simulink model "BLDCmotor_FOC_R2017b_fixdt"  (R2025a)
settings: Solver=FixedStepDiscrete  StartTime=0  StopTime=0.5  FixedStep=Ts  MaxStep=1e-6  RelTol=1e-6  AbsTol=1e-6  EnableMultiTasking=on
PreLoadFcn:
  | addpath(pwd);
  | addpath(genpath('01_Libraries'));
  | addpath(genpath('02_Figures'));
  | addpath(genpath('03_CreateParamTable'));
InitFcn:
  | init_model;
values from neighbouring files (symbols this model uses):
  a_cpr = 65535    [init_model.m]
  a_elecAngle = 60    [init_model.m]
  a_elecoffset = a_elecPeriod/12    (= 30)    [init_model.m]
  a_elecPeriod = 360    [init_model.m]
  a_fcpr = 1/65535    (= 1.52590218967e-05)    [init_model.m]
  a_mechoffset = a_elecoffset/n_polePairs    (= 5)    [init_model.m]
  a_phaAdvMax = 25    [init_model.m]
  b_angleMeasEna = 1    [init_model.m]
  b_cruiseCtrlEna = 0    [init_model.m]
  b_diagEna = 0    [init_model.m]
  b_fieldWeakEna = 0    [init_model.m]
  cf_currFilt = 0.692    [init_model.m]
  cf_idKi = Ki / (f_ctrl)    (= 0.00409061543436)    [init_model.m]
  cf_idKp = Kp    (= 0.0523598775598)    [init_model.m]
  cf_iqKi = Ki / (f_ctrl)    (= 0.00409061543436)    [init_model.m]
  cf_iqKiLimProt = 60 / (f_ctrl)    (= 0.00375)    [init_model.m]
  cf_iqKp = Kp    (= 0.0523598775598)    [init_model.m]
  cf_KbLimProt = Simulink.Parameter    [init_model.m]
  cf_nKi = 20.4 / (f_ctrl)    (= 0.001275)    [init_model.m]
  cf_nKiLimProt = 20 / (f_ctrl)    (= 0.00125)    [init_model.m]
  cf_nKp = 1.18    [init_model.m]
  cf_speedCoef = round(f_ctrl * a_mechAngle * (pi/180) * (30/pi))    [init_model.m]
  CTRL_FOC = 2    [init_model.m]
  CTRL_SIN = 1    [init_model.m]
  dV_openRate = 1000 / (f_ctrl)    (= 0.0625)    [init_model.m]
  dz_cntTrnsDetHi = 40    [init_model.m]
  dz_cntTrnsDetLo = 20    [init_model.m]
  ff_gain = ((r_motn / i_sca) * ((GD32_Vd_max_margin) / v_bus))    (= 0.338958333333)    [init_model.m]
  GD32_Vd_max_margin = GD32_Vd_max - V_margin    (= 1627)    [init_model.m]
  GD32_Vq_max_M1 = sqrt(GD32_Vd_max_margin^2 - GD32_Vq_max_XA.^2)    [init_model.m]
  i_max = i_max * i_sca    (= 500)    [init_model.m]
  id_fieldWeakMax = 5 * i_sca    (= 250)    [init_model.m]
  iq_maxSca_M1 = sqrt(1 - iq_maxSca_XA.^2)    [init_model.m]
  mcu_model = GD32F103    (= 1)    [init_model.m]
  n_commAcvLo = 15    [init_model.m]
  n_commDeacvHi = 30    [init_model.m]
  n_cruiseMotTgt = 0    [init_model.m]
  n_fieldWeakAuthHi = 300    [init_model.m]
  n_fieldWeakAuthLo = 100    [init_model.m]
  n_max = 1950    [init_model.m]
  n_polePairs = 6    [init_model.m]
  n_stdStillDet = 3    [init_model.m]
  OPEN_MODE = 0    [init_model.m]
  r_cos_M1 = cos((a_elecAngle_XA + a_elecPeriod/12)*(pi/180))    [init_model.m]
  r_errInpTgtThres = 600    [init_model.m]
  r_fieldWeakHi = 1000    [init_model.m]
  r_fieldWeakLo = 750    [init_model.m]
  r_motn = r_mot/2    (= 0.25)    [init_model.m]
  r_sin3PhaA_M1 = sin3Arm + A*r_sinPhaA_M1    [init_model.m]
  r_sin3PhaB_M1 = sin3Arm + A*r_sinPhaB_M1    [init_model.m]
  r_sin3PhaC_M1 = sin3Arm + A*r_sinPhaC_M1    [init_model.m]
  r_sin_M1 = sin((a_elecAngle_XA + a_elecPeriod/12)*(pi/180))    [init_model.m]
  SPD_MODE = 2    [init_model.m]
  STM32_Vd_max_margin = STM32_Vd_max - V_margin    (= 940)    [init_model.m]
  STM32_Vq_max_M1 = sqrt(STM32_Vd_max_margin^2 - STM32_Vq_max_XA.^2)    [init_model.m]
  t_errDequal = 1.80 * f_ctrl    (= 28800)    [init_model.m]
  t_errQual = 0.24 * f_ctrl    (= 3840)    [init_model.m]
  tgt_scale = 2047    [init_model.m]
  TRQ_MODE = 3    [init_model.m]
  Ts = 5e-6    (= 5e-06)    [init_model.m]
  Ts_ctrl = 6e-5    (= 6e-05)    [init_model.m]
  v_bus = 24    [init_model.m]
  vec_hallToPos = [0 2 0 1 4 3 5 0]    [init_model.m]
  VLT_MODE = 1    [init_model.m]
  z_commutMap_M1 = [-1 -1  0  1  1  0 ... (first row only)    [init_model.m]
  z_ctrlModReq = TRQ_MODE    (= 3)    [init_model.m]
  z_ctrlTypSel = CTRL_FOC    (= 2)    [init_model.m]
  z_maxCntRst = 2000    [init_model.m]
  z_selPhaCurMeasABC = 2    [init_model.m]
undefined symbols (not defined in the file or in its folder): BLDCmotor_FOC_R2017b_fixdt, DiscIntNeverNeededParam, DWORK0, DWORK1, DWORK2, DWORK3, powergui, spspowerguiLib
libraries: BLDC_controller_Lib x18, simulink x13, prociolib x6, eePwmGenerator x6, eePwmGeneratorMultilevel x3, mcbpositiondecoderlib x2, slpidlib x2, spsControlledVoltageSourceLib x1, spsMultimeterLib x1, spsPermanentMagnetSynchronousMachineLib x1, spsUniversalBridgeLib x1, spsVoltageMeasurementLib x1
(part 5 of 6)

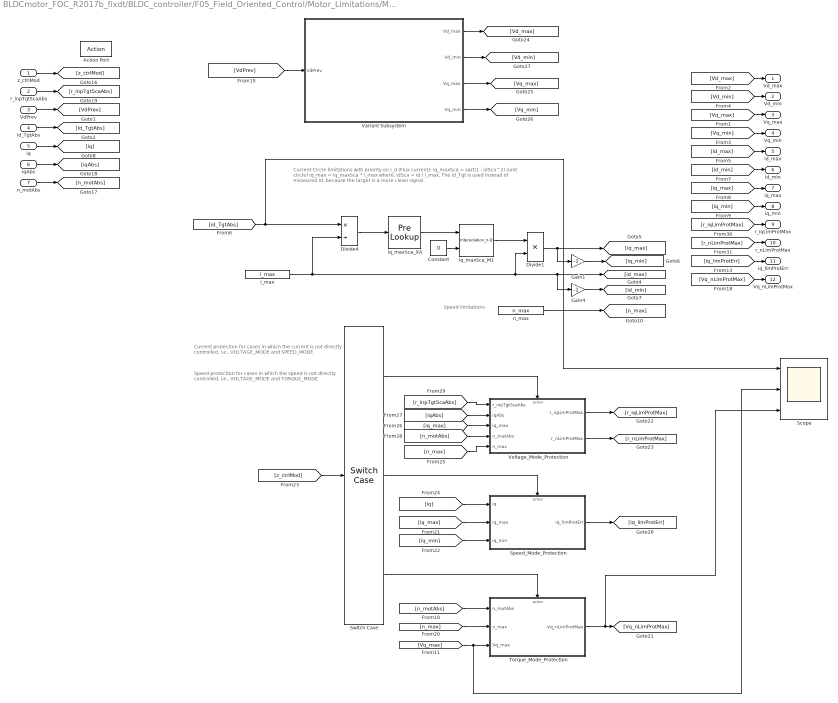
== system BLDCmotor_FOC_R2017b_fixdt/BLDC_controller/F05_Field_Oriented_Control/Motor_Limitations/Motor_Limitations_Enabled ==
  note: Current Circle limitations with priority on i_d (Flux current):
      | iq_maxSca = sqrt(1 - idSca^2) (unit circle)
      | iq_max = iq_maxSca * i_max
      |
      | where, idSca = id / i_max,
      |
      | The id_Tgt is used instead of measured id, because the target is a more clean signal.
  note: Speed limitations
  note: Current protection
      | for cases in which the current is not directly controlled, i.e., VOLTAGE_MODE and SPEED_MODE
  note: Speed protection
      | for cases in which the speed is not directly controlled, i.e., VOLTAGE_MODE and TORQUE_MODE
  z_ctrlMod : Inport
  r_inpTgtScaAbs : Inport  Port=2
  VdPrev : Inport  Port=3
  id_TgtAbs : Inport  Port=4
  iq : Inport  Port=5
  iqAbs : Inport  Port=6
  n_motAbs : Inport  Port=7
  Action Port : ActionPort  ActionPortLabel=if(u1 == CTRL_FOC)
  Constant : Constant  Value=0  OutDataTypeStr=int8
  Divide1 : Product  Inputs=**  OutDataTypeStr=fixdt(1,16,4)  RndMeth=Simplest
  Divide4 : Product  Inputs=*/  OutDataTypeStr=fixdt(0,16,16)  RndMeth=Simplest  SaturateOnIntegerOverflow=on
  Gain1 : Gain  Tag=struct('comment',struct('text','','placement',1),'logdata',struct('maxnumvals',inf,'plotchannels',[],'loggingmode',3,'channels',1),'output',struct('variable','','description','','name','$S_$B','width',1,'address','','max',NaN,'min',NaN,'class','default','type','CONTINUOUS','scaling','','lsb',1,'offset',0,'arb',0,'freeze',1,'unit','','autoscalingmode',1,'lowerheadroom',1,'upperheadroom',1,'headroomunit','bit','keepdatatype',1,'checkmin',0,'checkmax',0,'castoutput',0,'show',0),'gain',struct('variable','','description','','name','$S_$B_gain','width',1,'address','','max',NaN,'min',NaN,'class','default','type','CONTINUOUS','scaling','','lsb',1,'offset',0,'arb',0,'freeze',1,'unit','','keepdatatype',1,'value','1','scalar',0,'tolerance',1),'scalingvalid',0,'date',730486)  Gain=-1  RndMeth=Zero  OutDataTypeStr=Inherit: Same as input  ParamDataTypeStr=Inherit: Same as input
  Gain4 : Gain  Tag=struct('comment',struct('text','','placement',1),'logdata',struct('maxnumvals',inf,'plotchannels',[],'loggingmode',3,'channels',1),'output',struct('variable','','description','','name','$S_$B','width',1,'address','','max',NaN,'min',NaN,'class','default','type','CONTINUOUS','scaling','','lsb',1,'offset',0,'arb',0,'freeze',1,'unit','','autoscalingmode',1,'lowerheadroom',1,'upperheadroom',1,'headroomunit','bit','keepdatatype',1,'checkmin',0,'checkmax',0,'castoutput',0,'show',0),'gain',struct('variable','','description','','name','$S_$B_gain','width',1,'address','','max',NaN,'min',NaN,'class','default','type','CONTINUOUS','scaling','','lsb',1,'offset',0,'arb',0,'freeze',1,'unit','','keepdatatype',1,'value','1','scalar',0,'tolerance',1),'scalingvalid',0,'date',730486)  Gain=-1  RndMeth=Zero  OutDataTypeStr=Inherit: Same as input  ParamDataTypeStr=Inherit: Same as input
  Scope : Scope  NumInputPorts=3
      settings: ActiveDisplayYMinimum=-836.81756243429641  ActiveDisplayYMaximum=2890.0679339454637  DataLoggingVariableName=ScopeData6
  Speed_Mode_Protection : Subsystem
  Switch Case : SwitchCase  CaseConditions={VLT_MODE, SPD_MODE, TRQ_MODE}  ShowDefaultCase=off
  Torque_Mode_Protection : Subsystem
  Variant Subsystem : Subsystem  Variant=on  VariantActivationTime=code compile
  Voltage_Mode_Protection : Subsystem
  i_max : Constant  Value=i_max  OutDataTypeStr=fixdt(1,16,4)
  iq_maxSca_M1 : Interpolation_n-D  NumberOfTableDimensions=1  Table=iq_maxSca_M1  InterpMethod=Flat  ExtrapMethod=Clip  DiagnosticForOutOfRangeInput=Error  RemoveProtectionIndex=on  ValidIndexMayReachLast=on  OutDataTypeStr=fixdt(0,16,16)  InternalRulePriority=Speed  RndMeth=Simplest
      settings: InputPortMap=u0,u1
  iq_maxSca_XA : PreLookup  BreakpointsData=iq_maxSca_XA  OutputSelection=Index only  IndexSearchMethod=Evenly spaced points  BeginIndexSearchUsingPreviousIndexResult=on  UseLastBreakpoint=on  RemoveProtectionInput=on  DiagnosticForOutOfRangeInput=Warning  IndexDataTypeStr=uint8  FractionDataTypeStr=fixdt(0,8,6)  RndMeth=Simplest
  n_max : Constant  Value=n_max  OutDataTypeStr=Inherit: Inherit via back propagation
  Vd_max : Outport  InitialOutput=900  VectorParamsAs1DForOutWhenUnconnected=off
  Vd_min : Outport  Port=2  InitialOutput=-900  VectorParamsAs1DForOutWhenUnconnected=off
  Vq_max : Outport  Port=3  InitialOutput=900  VectorParamsAs1DForOutWhenUnconnected=off
  Vq_min : Outport  Port=4  InitialOutput=-900  VectorParamsAs1DForOutWhenUnconnected=off
  id_max : Outport  Port=5  InitialOutput=750  VectorParamsAs1DForOutWhenUnconnected=off
  id_min : Outport  Port=6  InitialOutput=-750  VectorParamsAs1DForOutWhenUnconnected=off
  iq_max : Outport  Port=7  InitialOutput=750  VectorParamsAs1DForOutWhenUnconnected=off
  iq_min : Outport  Port=8  InitialOutput=-750  VectorParamsAs1DForOutWhenUnconnected=off
  r_iqLimProtMax : Outport  Port=9  VectorParamsAs1DForOutWhenUnconnected=off
  r_nLimProtMax : Outport  Port=10  VectorParamsAs1DForOutWhenUnconnected=off
  iq_limProtErr : Outport  Port=11  VectorParamsAs1DForOutWhenUnconnected=off
  Vq_nLimProtMax : Outport  Port=12  VectorParamsAs1DForOutWhenUnconnected=off
  wires:
  [Vq_min] -> Vq_min/1
  [Vq_max] -> Vq_max/1
  VdPrev/1 -> [VdPrev]
  id_TgtAbs/1 -> [id_TgtAbs]
  [Vd_max] -> Vd_max/1
  [Vd_min] -> Vd_min/1
  Gain4/1 -> [id_min]
  i_max/1 -> Divide1/2, [id_max], Gain4/1, Divide4/2
  Divide4/1 -> iq_maxSca_XA/1
  Divide1/1 -> Gain1/1, [iq_max]
  Gain1/1 -> [iq_min]
  [id_min] -> id_min/1
  [id_max] -> id_max/1
  [iq_max] -> iq_max/1
  [iq_min] -> iq_min/1
  iq/1 -> [iq]
  [iq_limProtErr] -> iq_limProtErr/1
  n_max/1 -> [n_max]
  [Vq_nLimProtMax] -> Vq_nLimProtMax/1
  z_ctrlMod/1 -> [z_ctrlMod]
  [id_TgtAbs] -> Divide4/1, Scope/1
  iq_maxSca_M1/1 -> Divide1/1
  [z_ctrlMod] -> Switch Case/1
  Switch Case/1 -> Voltage_Mode_Protection/Action
  Switch Case/2 -> Speed_Mode_Protection/Action
  Switch Case/3 -> Torque_Mode_Protection/Action
  [n_max] -> Torque_Mode_Protection/2(n_max)
  [iq] -> Speed_Mode_Protection/1(iq)
  [iq_min] -> Speed_Mode_Protection/3(iq_min)
  [iq_max] -> Speed_Mode_Protection/2(iq_max)
  [n_max] -> Voltage_Mode_Protection/5(n_max)
  [iq_max] -> Voltage_Mode_Protection/3(iq_max)
  n_motAbs/1 -> [n_motAbs]
  iqAbs/1 -> [iqAbs]
  [iqAbs] -> Voltage_Mode_Protection/2(iqAbs)
  [n_motAbs] -> Voltage_Mode_Protection/4(n_motAbs)
  r_inpTgtScaAbs/1 -> [r_inpTgtScaAbs]
  [r_inpTgtScaAbs] -> Voltage_Mode_Protection/1(r_inpTgtScaAbs)
  [r_nLimProtMax] -> r_nLimProtMax/1
  [r_iqLimProtMax] -> r_iqLimProtMax/1
  Speed_Mode_Protection/1(iq_limProtErr) -> [iq_limProtErr]
  Torque_Mode_Protection/1(Vq_nLimProtMax) -> Scope/3, [Vq_nLimProtMax]
  Voltage_Mode_Protection/1(r_iqLimProtMax) -> [r_iqLimProtMax]
  Voltage_Mode_Protection/2(r_nLimProtMax) -> [r_nLimProtMax]
  [n_motAbs] -> Torque_Mode_Protection/1(n_motAbs)
  [Vq_max] -> Scope/2, Torque_Mode_Protection/3(Vq_max)
  iq_maxSca_XA/1 -> iq_maxSca_M1/1
  Variant Subsystem/3(Vq_max) -> [Vq_max]
  Variant Subsystem/4(Vq_min) -> [Vq_min]
  Variant Subsystem/1(Vd_max) -> [Vd_max]
  Variant Subsystem/2(Vd_min) -> [Vd_min]
  Constant/1 -> iq_maxSca_M1/2
  [VdPrev] -> Variant Subsystem/1(VdPrev)

== system BLDCmotor_FOC_R2017b_fixdt/BLDC_controller/F06_Control_Type_Management/SIN_Method/Final_Phase_Advance_Calculation ==
  note: Phase Advance / Field Weakening
  a_elecAngle : Inport
  z_dir : Inport  Port=2
  r_fieldWeak : Inport  Port=3
  Modulo_fixdt : BLDC_controller_Lib/Modulo_fixdt  SystemSampleTime=-1  VariantActivationTime=update diagram  EmptyChoice=off  PassThrough=off  PassThroughVariantControl=(default)  EmptyChoiceVariantControl=(default)  AllowFlexibleInterface=on  Latency=0  AutoFrameSizeCalculation=off
  Mux : Mux  Inputs=2
  Product2 : Product  RndMeth=Simplest  OutDataTypeStr=Inherit: Same as first input
  Scope : Scope  NumInputPorts=2
      settings: ActiveDisplayYMinimum=-45  ActiveDisplayYMaximum=405
  Sum3 : Sum  RndMeth=Simplest  OutDataTypeStr=Inherit: Same as first input
  Switch_PhaAdv : Switch  Criteria=u2 ~= 0  OutDataTypeStr=Inherit: Inherit via back propagation  RndMeth=Zero  SaturateOnIntegerOverflow=off  InputSameDT=off
  a_elecPeriod2 : Constant  Value=a_elecPeriod  OutDataTypeStr=Inherit: Inherit via back propagation
  b_fieldWeakEna : Constant  Value=b_fieldWeakEna  OutDataTypeStr=boolean
  a_elecAngleAdv : Outport  OutputWhenDisabled=reset  InitialOutput=0  VectorParamsAs1DForOutWhenUnconnected=off
  tag scope: a_elecAngle=global
  wires:
  [r_fieldWeak] -> Product2/1
  [z_dir] -> Product2/2
  z_dir/1 -> [z_dir]
  Mux/1 -> Scope/1
  Modulo_fixdt/1 -> Switch_PhaAdv/1
  [a_elecAngleAdv] -> a_elecAngleAdv/1
  [r_fieldWeak] -> Scope/2
  [a_elecAngle] -> Sum3/1
  a_elecPeriod2/1 -> Modulo_fixdt/2
  Sum3/1 -> Modulo_fixdt/1
  r_fieldWeak/1 -> [r_fieldWeak]
  a_elecAngle/1 -> [a_elecAngle]
  b_fieldWeakEna/1 -> Switch_PhaAdv/2
  Product2/1 -> Sum3/2
  [a_elecAngle] -> Mux/1
  [a_elecAngle] -> Switch_PhaAdv/3
  Switch_PhaAdv/1 -> [a_elecAngleAdv]
  [a_elecAngleAdv] -> Mux/2

== system BLDCmotor_FOC_R2017b_fixdt/BLDC_model_open1/powergui/EquivalentModel1/Gates ==
  Mux : Mux  Inputs=1
  gates : Outport  VectorParamsAs1DForOutWhenUnconnected=off
  wires:
  Mux/1 -> gates/1
  [T65_5867_7152151077466] -> Mux/1

== system BLDCmotor_FOC_R2017b_fixdt/BLDC_model_open1/powergui/EquivalentModel1/Sources ==
  Mux : Mux  Inputs=[6 2 1]
  u : Outport  VectorParamsAs1DForOutWhenUnconnected=off
  wires:
  Mux/1 -> u/1
  [T66_5829_6032809763487] -> Mux/1
  [T85_7797_12671394611787] -> Mux/2
  [T75_6799_9389895368155] -> Mux/3

== system BLDCmotor_FOC_R2017b_fixdt/BLDC_model_open1/powergui/EquivalentModel1/Status ==
  status : Inport
  Demux : Demux  Outputs=1
  tag scope: T67_6102_7976573094514=global
  wires:
  status/1 -> Demux/1
  Demux/1 -> [T67_6102_7976573094514]

== system BLDCmotor_FOC_R2017b_fixdt/BLDC_model_open1/powergui/EquivalentModel1/Yout ==
  v,i : Inport
  Demux : Demux  Outputs=[6 2 1 17]
  tag scope: T68_6201_8120743405540=global, T71_6502_9056880373131=global, T85_7792_12590097096297=global, gotomultimeterPSB=global
  wires:
  v,i/1 -> Demux/1
  Demux/1 -> [T68_6201_8120743405540]
  Demux/2 -> [T85_7792_12590097096297]
  Demux/3 -> [T71_6502_9056880373131]
  Demux/4 -> [gotomultimeterPSB]

== system BLDCmotor_FOC_R2017b_fixdt/BLDC_controller/F03_Control_Mode_Manager/F03_03_Input_Target_Synthesis/FOC_Control_Type/Variant Subsystem1 ==
  note: 1) Add Subsystem or Model blocks as valid variant choices.
      | 2) You cannot connect blocks at this level. At simulation, connectivity is automatically
      | determined, based on the active variant and port name matching.
  GD32F103 : Subsystem  TreatAsAtomicUnit=on  VariantControl=mcu_model == 1
  STM32F103 : Subsystem  TreatAsAtomicUnit=on  VariantControl=mcu_model == 0
  Vd_max_margin : Outport

== system BLDCmotor_FOC_R2017b_fixdt/BLDC_controller/F05_Field_Oriented_Control/Clarke_Park_Transform_Forward/Clarke_Transform/Clarke_PhasesAB ==
  note: Clarke Transform:
      | i_alpha = i_phaA
      | i_beta = ((1/sqrt(3))*i_phaA + (2/sqrt(3))*i_phaB)
  i_phaA : Inport
  i_phaB : Inport  Port=2
  Action Port : ActionPort  ActionPortLabel=if(u1 == 0)
  From : From  Commented=on  GotoTag=i_phaA
  From1 : From  Commented=on  GotoTag=i_phaB
  Gain2 : Gain  Tag=struct('comment',struct('text','','placement',1),'logdata',struct('maxnumvals',inf,'plotchannels',[],'loggingmode',3,'channels',1),'output',struct('variable','','description','','name','$S_$B','width',1,'address','','max',NaN,'min',NaN,'class','default','type','CONTINUOUS','scaling','','lsb',1,'offset',0,'arb',0,'freeze',1,'unit','','autoscalingmode',1,'lowerheadroom',1,'upperheadroom',1,'headroomunit','bit','keepdatatype',1,'checkmin',0,'checkmax',0,'castoutput',0,'show',0),'gain',struct('variable','','description','','name','$S_$B_gain','width',1,'address','','max',NaN,'min',NaN,'class','default','type','CONTINUOUS','scaling','','lsb',1,'offset',0,'arb',0,'freeze',1,'unit','','keepdatatype',1,'value','1','scalar',0,'tolerance',1),'scalingvalid',0,'date',730486)  Commented=on  Gain=2/sqrt(3)  RndMeth=Simplest  OutDataTypeStr=Inherit: Same as input
  Gain4 : Gain  Tag=struct('comment',struct('text','','placement',1),'logdata',struct('maxnumvals',inf,'plotchannels',[],'loggingmode',3,'channels',1),'output',struct('variable','','description','','name','$S_$B','width',1,'address','','max',NaN,'min',NaN,'class','default','type','CONTINUOUS','scaling','','lsb',1,'offset',0,'arb',0,'freeze',1,'unit','','autoscalingmode',1,'lowerheadroom',1,'upperheadroom',1,'headroomunit','bit','keepdatatype',1,'checkmin',0,'checkmax',0,'castoutput',0,'show',0),'gain',struct('variable','','description','','name','$S_$B_gain','width',1,'address','','max',NaN,'min',NaN,'class','default','type','CONTINUOUS','scaling','','lsb',1,'offset',0,'arb',0,'freeze',1,'unit','','keepdatatype',1,'value','1','scalar',0,'tolerance',1),'scalingvalid',0,'date',730486)  Commented=on  Gain=1/sqrt(3)  RndMeth=Simplest  OutDataTypeStr=Inherit: Same as input
  Signal Conversion2 : SignalConversion  Commented=on  OverrideOpt=off
  Sum1 : Sum  Commented=on  OutDataTypeStr=Inherit: Inherit via back propagation  RndMeth=Simplest  SaturateOnIntegerOverflow=on
  a_plus_2b : Sum  Inputs=+++  RndMeth=Simplest  OutDataTypeStr=Inherit: Same as first input
  one_by_sqrt3 : Gain  Gain=1/sqrt(3)  RndMeth=Simplest  OutDataTypeStr=Inherit: Same as input
  i_alphaAB : Outport  VectorParamsAs1DForOutWhenUnconnected=off
  i_betaAB : Outport  Port=2  VectorParamsAs1DForOutWhenUnconnected=off
  wires:
  Gain4/1 -> Sum1/1
  Signal Conversion2/1 -> ?
  Sum1/1 -> ?
  From1/1 -> Gain2/1
  Gain2/1 -> Sum1/2
  From/1 -> Signal Conversion2/1, Gain4/1
  a_plus_2b/1 -> one_by_sqrt3/1
  one_by_sqrt3/1 -> i_betaAB/1
  i_phaA/1 -> i_alphaAB/1, a_plus_2b/1
  i_phaB/1 -> a_plus_2b/2, a_plus_2b/3

== system BLDCmotor_FOC_R2017b_fixdt/BLDC_controller/F05_Field_Oriented_Control/Clarke_Park_Transform_Forward/Clarke_Transform/Clarke_PhasesAC ==
  note: Clarke Transform:
      | i_alpha = i_phaA
      | i_beta = (-(1/sqrt(3))*i_phaA - (2/sqrt(3))*i_phaC)
  i_phaA : Inport
  i_phaC : Inport  Port=2
  Action Port : ActionPort  ActionPortLabel=else
  From : From  Commented=on  GotoTag=i_phaA
  From1 : From  Commented=on  GotoTag=i_phaC
  Gain2 : Gain  Tag=struct('comment',struct('text','','placement',1),'logdata',struct('maxnumvals',inf,'plotchannels',[],'loggingmode',3,'channels',1),'output',struct('variable','','description','','name','$S_$B','width',1,'address','','max',NaN,'min',NaN,'class','default','type','CONTINUOUS','scaling','','lsb',1,'offset',0,'arb',0,'freeze',1,'unit','','autoscalingmode',1,'lowerheadroom',1,'upperheadroom',1,'headroomunit','bit','keepdatatype',1,'checkmin',0,'checkmax',0,'castoutput',0,'show',0),'gain',struct('variable','','description','','name','$S_$B_gain','width',1,'address','','max',NaN,'min',NaN,'class','default','type','CONTINUOUS','scaling','','lsb',1,'offset',0,'arb',0,'freeze',1,'unit','','keepdatatype',1,'value','1','scalar',0,'tolerance',1),'scalingvalid',0,'date',730486)  Commented=on  Gain=2/sqrt(3)  RndMeth=Zero  OutDataTypeStr=Inherit: Same as input
  Gain4 : Gain  Tag=struct('comment',struct('text','','placement',1),'logdata',struct('maxnumvals',inf,'plotchannels',[],'loggingmode',3,'channels',1),'output',struct('variable','','description','','name','$S_$B','width',1,'address','','max',NaN,'min',NaN,'class','default','type','CONTINUOUS','scaling','','lsb',1,'offset',0,'arb',0,'freeze',1,'unit','','autoscalingmode',1,'lowerheadroom',1,'upperheadroom',1,'headroomunit','bit','keepdatatype',1,'checkmin',0,'checkmax',0,'castoutput',0,'show',0),'gain',struct('variable','','description','','name','$S_$B_gain','width',1,'address','','max',NaN,'min',NaN,'class','default','type','CONTINUOUS','scaling','','lsb',1,'offset',0,'arb',0,'freeze',1,'unit','','keepdatatype',1,'value','1','scalar',0,'tolerance',1),'scalingvalid',0,'date',730486)  Commented=on  Gain=1/sqrt(3)  RndMeth=Zero  OutDataTypeStr=Inherit: Same as input
  Goto13 : Goto  Commented=on  GotoTag=i_phaC
  Goto15 : Goto  Commented=on  GotoTag=i_phaA
  Signal Conversion2 : SignalConversion  Commented=on  OverrideOpt=off
  Sum1 : Sum  Commented=on  Inputs=--  OutDataTypeStr=Inherit: Inherit via back propagation  RndMeth=Simplest  SaturateOnIntegerOverflow=on
  a_plus_2b : Sum  Inputs=---  RndMeth=Simplest  OutDataTypeStr=Inherit: Same as first input
  one_by_sqrt3 : Gain  Gain=1/sqrt(3)  RndMeth=Simplest  OutDataTypeStr=Inherit: Same as input
  i_alphaAC : Outport  VectorParamsAs1DForOutWhenUnconnected=off
  i_betaAC : Outport  Port=2  VectorParamsAs1DForOutWhenUnconnected=off
  wires:
  a_plus_2b/1 -> one_by_sqrt3/1
  i_phaA/1 -> i_alphaAC/1, a_plus_2b/1
  i_phaC/1 -> a_plus_2b/2, a_plus_2b/3
  one_by_sqrt3/1 -> i_betaAC/1
  From1/1 -> Gain2/1
  Sum1/1 -> ?
  Gain4/1 -> Sum1/1
  Signal Conversion2/1 -> ?
  Gain2/1 -> Sum1/2
  From/1 -> Gain4/1, Signal Conversion2/1

== system BLDCmotor_FOC_R2017b_fixdt/BLDC_controller/F05_Field_Oriented_Control/Clarke_Park_Transform_Forward/Clarke_Transform/Clarke_PhasesBC ==
  note: Clarke Transform:
      | i_alpha = - i_phaB - i_phaC
      | i_beta = (1/sqrt(3)) * (i_phaB - i_phaC)
  i_phaB : Inport
  i_phaC : Inport  Port=2
  Action Port : ActionPort  ActionPortLabel=elseif(u1 == 1)
  Gain2 : Gain  Tag=struct('comment',struct('text','','placement',1),'logdata',struct('maxnumvals',inf,'plotchannels',[],'loggingmode',3,'channels',1),'output',struct('variable','','description','','name','$S_$B','width',1,'address','','max',NaN,'min',NaN,'class','default','type','CONTINUOUS','scaling','','lsb',1,'offset',0,'arb',0,'freeze',1,'unit','','autoscalingmode',1,'lowerheadroom',1,'upperheadroom',1,'headroomunit','bit','keepdatatype',1,'checkmin',0,'checkmax',0,'castoutput',0,'show',0),'gain',struct('variable','','description','','name','$S_$B_gain','width',1,'address','','max',NaN,'min',NaN,'class','default','type','CONTINUOUS','scaling','','lsb',1,'offset',0,'arb',0,'freeze',1,'unit','','keepdatatype',1,'value','1','scalar',0,'tolerance',1),'scalingvalid',0,'date',730486)  Gain=1/sqrt(3)  RndMeth=Zero  OutDataTypeStr=Inherit: Same as input
  Sum1 : Sum  Inputs=--  OutDataTypeStr=Inherit: Inherit via back propagation  RndMeth=Simplest  SaturateOnIntegerOverflow=on
  Sum3 : Sum  Inputs=+-  OutDataTypeStr=Inherit: Inherit via back propagation  RndMeth=Simplest  SaturateOnIntegerOverflow=on
  i_alphaBC : Outport  VectorParamsAs1DForOutWhenUnconnected=off
  i_betaBC : Outport  Port=2  VectorParamsAs1DForOutWhenUnconnected=off
  wires:
  [i_phaC] -> Sum1/2
  [i_phaB] -> Sum1/1
  [i_phaC] -> Sum3/2
  Gain2/1 -> i_betaBC/1
  Sum3/1 -> Gain2/1
  [i_phaB] -> Sum3/1
  Sum1/1 -> i_alphaBC/1
  i_phaB/1 -> [i_phaB]
  i_phaC/1 -> [i_phaC]

== system BLDCmotor_FOC_R2017b_fixdt/BLDC_controller/F05_Field_Oriented_Control/FOC/FOC_Enabled/Open_Mode ==
  note: Just copy the target which will be reduced to 0 in the Input_Target_Sythesis function.
  r_inpTgtSca : Inport
  Action Port : ActionPort  ActionPortLabel=default:
  Vq_Open : Outport  VectorParamsAs1DForOutWhenUnconnected=off
  wires:
  r_inpTgtSca/1 -> Vq_Open/1

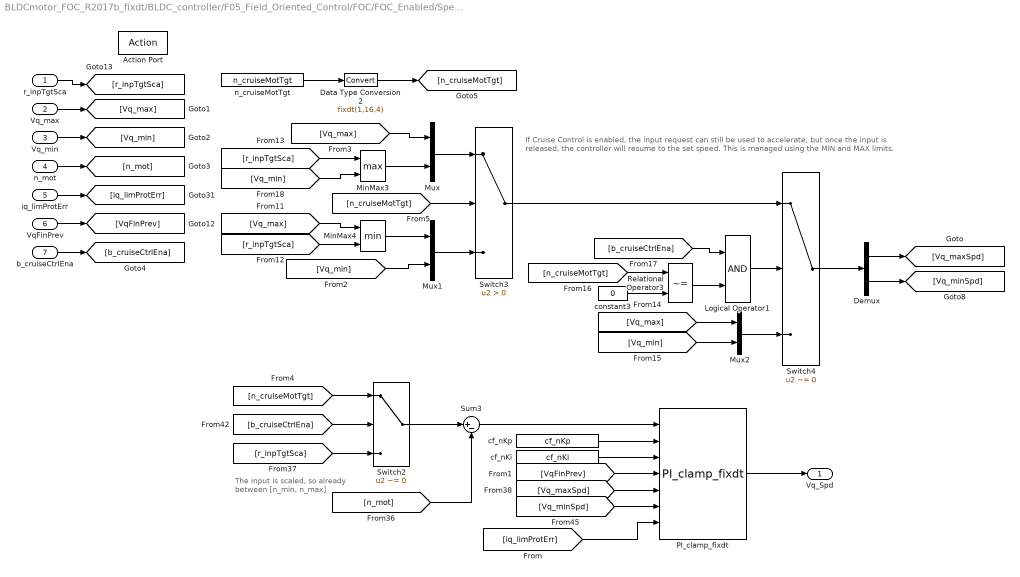
== system BLDCmotor_FOC_R2017b_fixdt/BLDC_controller/F05_Field_Oriented_Control/FOC/FOC_Enabled/Speed_Mode ==
  note: The input is scaled, so already between [n_min, n_max]
  note: If Cruise Control is enabled, the input request can still be used to accelerate, but once the input is released, the controller will resume to the set speed. This is managed using the MIN and MAX limits.
  r_inpTgtSca : Inport
  Vq_max : Inport  Port=2
  Vq_min : Inport  Port=3
  n_mot : Inport  Port=4
  iq_limProtErr : Inport  Port=5
  VqFinPrev : Inport  Port=6
  b_cruiseCtrlEna : Inport  Port=7
  Action Port : ActionPort  InitializeStates=reset  ActionPortLabel=case [ 2 ]:
  Data Type Conversion2 : DataTypeConversion  OutDataTypeStr=fixdt(1,16,4)  SaturateOnIntegerOverflow=off  RndMeth=Floor
  Demux : Demux  Outputs=2
  Logical Operator1 : Logic  AllPortsSameDT=off  OutDataTypeStr=boolean
  MinMax3 : MinMax  Function=max  Inputs=2
  MinMax4 : MinMax  Inputs=2
  Mux : Mux  Inputs=2
  Mux1 : Mux  Inputs=2
  Mux2 : Mux  Inputs=2
  PI_clamp_fixdt : BLDC_controller_Lib/PI_clamp_fixdt  SystemSampleTime=-1  VariantActivationTime=update diagram  EmptyChoice=off  PassThrough=off  PassThroughVariantControl=(default)  EmptyChoiceVariantControl=(default)  AllowFlexibleInterface=on  Latency=0  AutoFrameSizeCalculation=off
  Relational Operator3 : RelationalOperator  Operator=~=  OutDataTypeStr=boolean  RndMeth=Simplest  InputSameDT=off
  Sum3 : Sum  Inputs=|+-  RndMeth=Simplest  SaturateOnIntegerOverflow=on
  Switch2 : Switch  Criteria=u2 ~= 0  OutDataTypeStr=Inherit: Inherit via back propagation  RndMeth=Zero  SaturateOnIntegerOverflow=off  InputSameDT=off
  Switch3 : Switch  Criteria=u2 > Threshold  OutDataTypeStr=Inherit: Inherit via back propagation  RndMeth=Zero  SaturateOnIntegerOverflow=off  InputSameDT=off
  Switch4 : Switch  Criteria=u2 ~= 0  OutDataTypeStr=Inherit: Inherit via back propagation  RndMeth=Zero  SaturateOnIntegerOverflow=off  InputSameDT=off
  cf_nKi : Constant  Value=cf_nKi  VectorParams1D=off  OutDataTypeStr=fixdt(0,16,16)
  cf_nKp : Constant  Value=cf_nKp  OutDataTypeStr=fixdt(0,16,12)
  constant3 : Constant  Value=0  OutDataTypeStr=Inherit: Inherit via back propagation
  n_cruiseMotTgt : Constant  Value=n_cruiseMotTgt  OutDataTypeStr=int16
  Vq_Spd : Outport  VectorParamsAs1DForOutWhenUnconnected=off
  wires:
  cf_nKi/1 -> PI_clamp_fixdt/3
  cf_nKp/1 -> PI_clamp_fixdt/2
  [n_mot] -> Sum3/2
  Sum3/1 -> PI_clamp_fixdt/1
  r_inpTgtSca/1 -> [r_inpTgtSca]
  Vq_max/1 -> [Vq_max]
  Vq_min/1 -> [Vq_min]
  n_mot/1 -> [n_mot]
  iq_limProtErr/1 -> [iq_limProtErr]
  [iq_limProtErr] -> PI_clamp_fixdt/7
  [Vq_minSpd] -> PI_clamp_fixdt/6
  [Vq_maxSpd] -> PI_clamp_fixdt/5
  VqFinPrev/1 -> [VqFinPrev]
  [b_cruiseCtrlEna] -> Switch2/2
  [r_inpTgtSca] -> Switch2/3
  Switch2/1 -> Sum3/1
  b_cruiseCtrlEna/1 -> [b_cruiseCtrlEna]
  PI_clamp_fixdt/1 -> Vq_Spd/1
  n_cruiseMotTgt/1 -> Data Type Conversion2/1
  [n_cruiseMotTgt] -> Switch2/1
  Data Type Conversion2/1 -> [n_cruiseMotTgt]
  Logical Operator1/1 -> Switch4/2
  MinMax4/1 -> Mux1/1
  [Vq_max] -> MinMax4/1
  Mux/1 -> Switch3/1
  MinMax3/1 -> Mux/2
  [n_cruiseMotTgt] -> Relational Operator3/1
  [b_cruiseCtrlEna] -> Logical Operator1/1
  Relational Operator3/1 -> Logical Operator1/2
  constant3/1 -> Relational Operator3/2
  [Vq_max] -> Mux2/1
  Switch3/1 -> Switch4/1
  [Vq_min] -> Mux2/2
  [Vq_min] -> MinMax3/2
  Mux1/1 -> Switch3/3
  Mux2/1 -> Switch4/3
  [r_inpTgtSca] -> MinMax3/1
  [Vq_max] -> Mux/1
  [r_inpTgtSca] -> MinMax4/2
  [n_cruiseMotTgt] -> Switch3/2
  [Vq_min] -> Mux1/2
  Switch4/1 -> Demux/1
  Demux/1 -> [Vq_maxSpd]
  Demux/2 -> [Vq_minSpd]
  [VqFinPrev] -> PI_clamp_fixdt/4

== system BLDCmotor_FOC_R2017b_fixdt/BLDC_controller/F05_Field_Oriented_Control/FOC/FOC_Enabled/Torque_Mode ==
  r_inpTgtSca : Inport
  Vq_max : Inport  Port=2
  Vq_min : Inport  Port=3
  iq : Inport  Port=4
  iq_max : Inport  Port=5
  iq_min : Inport  Port=6
  Vq_nLimProtMax : Inport  Port=7
  VqFinPrev : Inport  Port=8
  Action Port : ActionPort  InitializeStates=reset  ActionPortLabel=case [ 3 ]:
  Constant : Constant  Value=0  OutDataTypeStr=Inherit: Inherit via back propagation
  FOC TQ PI : Scope  NumInputPorts=8
      settings: ActiveDisplayYMinimum=33.718101792372977  ActiveDisplayYMaximum=1221.9112315530967  DataLoggingVariableName=ScopeData5
  Gain4 : Gain  Tag=struct('comment',struct('text','','placement',1),'logdata',struct('maxnumvals',inf,'plotchannels',[],'loggingmode',3,'channels',1),'output',struct('variable','','description','','name','$S_$B','width',1,'address','','max',NaN,'min',NaN,'class','default','type','CONTINUOUS','scaling','','lsb',1,'offset',0,'arb',0,'freeze',1,'unit','','autoscalingmode',1,'lowerheadroom',1,'upperheadroom',1,'headroomunit','bit','keepdatatype',1,'checkmin',0,'checkmax',0,'castoutput',0,'show',0),'gain',struct('variable','','description','','name','$S_$B_gain','width',1,'address','','max',NaN,'min',NaN,'class','default','type','CONTINUOUS','scaling','','lsb',1,'offset',0,'arb',0,'freeze',1,'unit','','keepdatatype',1,'value','1','scalar',0,'tolerance',1),'scalingvalid',0,'date',730486)  Gain=-1  RndMeth=Zero  OutDataTypeStr=Inherit: Same as input  ParamDataTypeStr=Inherit: Same as input
  MinMax1 : MinMax  Inputs=2  OutDataTypeStr=Inherit: Inherit via back propagation
  MinMax2 : MinMax  Function=max  Inputs=2  OutDataTypeStr=Inherit: Inherit via back propagation
  PI Controller : slpidlib/PID Controller  Commented=on  Controller=PI  Form=Parallel  TimeDomain=Discrete-time  UseExternalTs=on  SampleTime=-1  IntegratorMethod=Forward Euler  FilterMethod=Forward Euler  ControllerParametersSource=external  P=0.6  I=0.05  UseKiTs=on  D=0  UseExternalDerivativeSource=off  N=100  UseFilter=on  TunerSelectOption=Transfer Function Based (PID Tuner App)  ZeroCross=off  InitialConditionSource=external  InitialConditionForIntegrator=0  InitialConditionForFilter=0  DifferentiatorICPrevScaledInput=0  ExternalReset=none  TrackingMode=off  Kt=1  LimitOutput=on  SatLimitsSource=external  UpperSaturationLimit=1  LowerSaturationLimit=-1  LinearizeAsGain=on  AntiWindupMode=clamping  Kb=1  LimitIntegrator=off  UpperIntegratorSaturationLimit=inf  LowerIntegratorSaturationLimit=-inf  RndMeth=Simplest  SaturateOnIntegerOverflow=on  POutMin=[]  POutMax=[]  IOutMin=[]  IOutMax=[]  DOutMin=[]  DOutMax=[]  NOutMin=[]  NOutMax=[]  SumOutMin=[]  SumOutMax=[]  SaturationOutDataTypeStr=Inherit: Inherit via back propagation  SaturationOutMin=[]  SaturationOutMax=[]  PParamMin=[]  PParamMax=[]  IParamMin=[]  IParamMax=[]  DParamMin=[]  DParamMax=[]  NParamMin=[]  NParamMax=[]  KbParamMin=[]  KbParamMax=[]  KtParamMin=[]  KtParamMax=[]  KbOutMin=[]  KbOutMax=[]  KtOutMin=[]  KtOutMax=[]  IntegratorOutMin=[]  IntegratorOutMax=[]  FilterOutMin=[]  FilterOutMax=[]  SumI1OutMin=[]  SumI1OutMax=[]  SumI2OutMin=[]  SumI2OutMax=[]  SumI3OutMin=[]  SumI3OutMax=[]  SumI4OutMin=[]  SumI4OutMax=[]  SumDOutMin=[]  SumDOutMax=[]  DifferentiatorOutMin=[]  DifferentiatorOutMax=[]  FilterDiffOutCoefMin=[]  FilterDiffOutCoefMax=[]  ReciprocalOutMin=[]  ReciprocalOutMax=[]  SumDenOutMin=[]  SumDenOutMax=[]  SumNumOutMin=[]  SumNumOutMax=[]  DivideOutMin=[]  DivideOutMax=[]  UdiffTsProdOutMin=[]  UdiffTsProdOutMax=[]  NTsProdOutMin=[]  NTsProdOutMax=[]  UintegralTsProdOutMin=[]  UintegralTsProdOutMax=[]  UngainTsProdOutMin=[]  UngainTsProdOutMax=[]  ClampingZeroOutDataTypeStr=Inherit: Inherit via back propagation  ClampingZeroOutMin=[]  ClampingZeroOutMax=[]  FilterDenConstantOutDataTypeStr=Inherit: Inherit via back propagation  FilterDenConstantOutMin=[]  FilterDenConstantOutMax=[]  PCopyOutDataTypeStr=Inherit: Inherit via back propagation  PCopyOutMin=[]  PCopyOutMax=[]  NCopyOutDataTypeStr=Inherit: Inherit via back propagation  NCopyOutMin=[]  NCopyOutMax=[]  IntegratorContinuousStateAttributes=''  IntegratorStateMustResolveToSignalObject=off  IntegratorRTWStateStorageClass=Auto  FilterContinuousStateAttributes=''  FilterStateMustResolveToSignalObject=off  FilterRTWStateStorageClass=Auto  ParallelPVariant=ExternalParameters  IdealPVariant=Disabled  IVariant=ExternalParameters  DVariant=Disabled  IntegratorVariant=Discrete  SatVariant=External  AWVariant=DiscClampingParallel  PCopyVariant=Disabled  TRVariant=Disabled  FdbkBlocksVariant=Forward  IdealPFdbkVariant=Disabled  SatFdbkVariant=Disabled  DerivativeFilterVariant=Disabled  NVariant=Disabled  NCopyVariant=Disabled_SignalSpec  FilterICVariant=Disabled  IntegratorICVariant=ExternalICs  ExternalResetVariant=Disabled  TRSumVariant=Passthrough  SumFdbkVariant=Disabled  SumVariant=Sum_PI  TsampFilterVariant=InternalTs  TsampNgainVariant=Passthrough  TsampIntegralVariant=Passthrough  ExternalSaturationOutDataTypeStr=Inherit: Same as second input  DerivativeSourceVariant=Disabled  PreIntVariant=InternalPreInt
      settings: LibrarySourceBlock=mcblib/Controls/Controllers/PI Controller
  PI_clamp_fixdtFF : Subsystem  TreatAsAtomicUnit=on
      settings: RTWFcnNameOpts=Use subsystem name
      mask Display: disp('PI(z)')
  Saturation Dynamic1 : simulink/Discontinuities/Saturation Dynamic  OutMin=[]  OutMax=[]  OutDataTypeStr=Inherit: Same as second input  OutDataType=fixdt(1, 16)  OutScaling=2^-10  DoSatur=off
  Signal Conversion2 : SignalConversion  OverrideOpt=off
  Sum2 : Sum  Inputs=|+-  RndMeth=Simplest  SaturateOnIntegerOverflow=on
  Variant Subsystem : Subsystem  Commented=on  Variant=on  VariantActivationTime=code compile
  cf_iqKi1 : Constant  Value=cf_iqKi  OutDataTypeStr=fixdt(0,16,16)
  cf_iqKp1 : Constant  Value=cf_iqKp  OutDataTypeStr=fixdt(0,16,13)
  Vq_Trq : Outport  VectorParamsAs1DForOutWhenUnconnected=off
  wires:
  Vq_max/1 -> [Vq_max]
  r_inpTgtSca/1 -> [r_inpTgtSca]
  Vq_min/1 -> [Vq_min]
  iq/1 -> [iq]
  iq_min/1 -> [iq_min]
  iq_max/1 -> [iq_max]
  Vq_nLimProtMax/1 -> [Vq_nLimProtMax]
  [iq_max] -> Saturation Dynamic1/1
  [iq_min] -> Saturation Dynamic1/3
  Sum2/1 -> PI_clamp_fixdtFF/1(err), FOC TQ PI/6
  [iq] -> FOC TQ PI/5, Sum2/2
  [Vq_minTrq] -> PI_clamp_fixdtFF/6(satMin), FOC TQ PI/4
  [Vq_maxTrq] -> PI_clamp_fixdtFF/5(satMax), FOC TQ PI/3
  [Vq_nLimProtMax] -> MinMax1/2, Gain4/1
  [Vq_max] -> MinMax1/1
  Gain4/1 -> MinMax2/1
  [Vq_min] -> MinMax2/2
  MinMax1/1 -> [Vq_maxTrq]
  MinMax2/1 -> [Vq_minTrq]
  [VqFinPrev] -> PI_clamp_fixdtFF/4(init), FOC TQ PI/2
  cf_iqKp1/1 -> PI_clamp_fixdtFF/2(P)
  cf_iqKi1/1 -> PI_clamp_fixdtFF/3(I)
  [r_inpTgtSca] -> Saturation Dynamic1/2
  Signal Conversion2/1 -> Vq_Trq/1, FOC TQ PI/8
  Constant/1 -> PI_clamp_fixdtFF/7(ext_limProt)
  PI_clamp_fixdtFF/1(out) -> FOC TQ PI/7, Signal Conversion2/1
  VqFinPrev/1 -> [VqFinPrev]
  Saturation Dynamic1/1 -> PI_clamp_fixdtFF/8(FeedForward), FOC TQ PI/1, Sum2/1

== system BLDCmotor_FOC_R2017b_fixdt/BLDC_controller/F05_Field_Oriented_Control/FOC/FOC_Enabled/Vd_Calculation ==
  id_TgtAbs : Inport
  id : Inport  Port=2
  Vd_max : Inport  Port=3
  Vd_min : Inport  Port=4
  id_max : Inport  Port=5
  id_min : Inport  Port=6
  Action Port : ActionPort  InitializeStates=reset  ActionPortLabel=if(u1 ~= 0)
  FOC VD : Scope  NumInputPorts=3
      settings: ActiveDisplayYMinimum=-1490.0965469412238  ActiveDisplayYMaximum=1096.0505036477102  DataLoggingVariableName=ScopeData3
  PI_clamp_fixdt : BLDC_controller_Lib/PI_clamp_fixdt  Commented=on  SystemSampleTime=-1  VariantActivationTime=update diagram  EmptyChoice=off  PassThrough=off  PassThroughVariantControl=(default)  EmptyChoiceVariantControl=(default)  AllowFlexibleInterface=on  Latency=0  AutoFrameSizeCalculation=off
  PI_clamp_fixdtFF : Subsystem  TreatAsAtomicUnit=on
      settings: RTWFcnNameOpts=Use subsystem name
      mask Display: disp('PI(z)')
  Saturation Dynamic : simulink/Discontinuities/Saturation Dynamic  OutMin=[]  OutMax=[]  OutDataTypeStr=Inherit: Same as second input  OutDataType=fixdt(1, 16)  OutScaling=2^-10  DoSatur=off
  Sum3 : Sum  Inputs=|+-  RndMeth=Simplest  SaturateOnIntegerOverflow=on
  cf_idKi2 : Constant  Value=cf_idKi  OutDataTypeStr=fixdt(0,16,16)
  cf_idKp2 : Constant  Value=cf_idKp  OutDataTypeStr=fixdt(0,16,13)
  constant1 : Constant  Value=0  OutDataTypeStr=Inherit: Inherit via back propagation
  constant2 : Constant  Value=0  OutDataTypeStr=Inherit: Inherit via back propagation
  toNegative : Gain  Tag=struct('comment',struct('text','','placement',1),'logdata',struct('maxnumvals',inf,'plotchannels',[],'loggingmode',3,'channels',1),'output',struct('variable','','description','','name','$S_$B','width',1,'address','','max',NaN,'min',NaN,'class','default','type','CONTINUOUS','scaling','','lsb',1,'offset',0,'arb',0,'freeze',1,'unit','','autoscalingmode',1,'lowerheadroom',1,'upperheadroom',1,'headroomunit','bit','keepdatatype',1,'checkmin',0,'checkmax',0,'castoutput',0,'show',0),'gain',struct('variable','','description','','name','$S_$B_gain','width',1,'address','','max',NaN,'min',NaN,'class','default','type','CONTINUOUS','scaling','','lsb',1,'offset',0,'arb',0,'freeze',1,'unit','','keepdatatype',1,'value','1','scalar',0,'tolerance',1),'scalingvalid',0,'date',730486)  Gain=-1  RndMeth=Zero  OutDataTypeStr=Inherit: Same as input  ParamDataTypeStr=Inherit: Same as input
  Vd : Outport  VectorParamsAs1DForOutWhenUnconnected=off
  wires:
  [id] -> Sum3/2
  [id_TgtAbs] -> toNegative/1
  id_TgtAbs/1 -> [id_TgtAbs]
  id/1 -> [id]
  Vd_min/1 -> [Vd_min]
  Vd_max/1 -> [Vd_max]
  id_max/1 -> [id_max]
  id_min/1 -> [id_min]
  [id_max] -> Saturation Dynamic/1
  [id_min] -> Saturation Dynamic/3
  Sum3/1 -> PI_clamp_fixdtFF/1(err), FOC VD/2
  [Vd_min] -> PI_clamp_fixdtFF/6(satMin)
  [Vd_max] -> PI_clamp_fixdtFF/5(satMax)
  constant2/1 -> PI_clamp_fixdtFF/4(init)
  toNegative/1 -> Saturation Dynamic/2
  cf_idKi2/1 -> PI_clamp_fixdtFF/3(I)
  cf_idKp2/1 -> PI_clamp_fixdtFF/2(P)
  Saturation Dynamic/1 -> PI_clamp_fixdtFF/8(FeedForward), FOC VD/1, Sum3/1
  PI_clamp_fixdtFF/1(out) -> FOC VD/3, Vd/1
  constant1/1 -> PI_clamp_fixdtFF/7(ext_limProt)

== system BLDCmotor_FOC_R2017b_fixdt/BLDC_controller/F05_Field_Oriented_Control/FOC/FOC_Enabled/Voltage_Mode ==
  r_inpTgtSca : Inport
  r_inpTgtScaAbs : Inport  Port=2
  Vq_max : Inport  Port=3
  Vq_min : Inport  Port=4
  r_iqLimProtMax : Inport  Port=5
  r_nLimProtMax : Inport  Port=6
  Action Port : ActionPort  InitializeStates=reset  ActionPortLabel=case [ 1 ]:
  Divide1 : Product  Inputs=**  RndMeth=Simplest  OutDataTypeStr=Inherit: Same as first input
  MinMax : MinMax  Inputs=3
  Saturation Dynamic1 : simulink/Discontinuities/Saturation Dynamic  OutMin=[]  OutMax=[]  OutDataTypeStr=Inherit: Same as second input  OutDataType=fixdt(1, 16)  OutScaling=2^-10  DoSatur=off
  SignDeltaU2 : Signum  DisableCoverage=on
  Signal Conversion2 : SignalConversion  OverrideOpt=off
  Vq_Vlt : Outport  VectorParamsAs1DForOutWhenUnconnected=off
  wires:
  r_inpTgtSca/1 -> [r_inpTgtSca]
  [Vq_min] -> Saturation Dynamic1/3
  [Vq_max] -> Saturation Dynamic1/1
  Vq_max/1 -> [Vq_max]
  Vq_min/1 -> [Vq_min]
  r_iqLimProtMax/1 -> [r_iqLimProtMax]
  r_nLimProtMax/1 -> [r_nLimProtMax]
  Signal Conversion2/1 -> Vq_Vlt/1
  Saturation Dynamic1/1 -> Signal Conversion2/1
  [r_nLimProtMax] -> MinMax/3
  r_inpTgtScaAbs/1 -> [r_inpTgtScaAbs]
  [r_inpTgtScaAbs] -> MinMax/1
  [r_inpTgtSca] -> SignDeltaU2/1
  MinMax/1 -> Divide1/1
  SignDeltaU2/1 -> Divide1/2
  Divide1/1 -> Saturation Dynamic1/2
  [r_iqLimProtMax] -> MinMax/2

== system BLDCmotor_FOC_R2017b_fixdt/BLDC_controller/F05_Field_Oriented_Control/Motor_Limitations/Motor_Limitations_Enabled/Speed_Mode_Protection ==
  iq : Inport
  iq_max : Inport  Port=2
  iq_min : Inport  Port=3
  Action Port : ActionPort  ActionPortLabel=case [ 2 ]:
  Divide1 : Product  Inputs=**  OutDataTypeStr=fixdt(1,32,20)  RndMeth=Simplest
  Saturation Dynamic : simulink/Discontinuities/Saturation Dynamic  OutMin=[]  OutMax=[]  OutDataTypeStr=Inherit: Same as second input  OutDataType=fixdt(1, 16)  OutScaling=2^-10  DoSatur=off
  Sum3 : Sum  Inputs=|+-  RndMeth=Simplest
  cf_iqKiLimProt : Constant  Value=cf_iqKiLimProt  OutDataTypeStr=fixdt(0,16,16)
  iq_limProtErr : Outport  InitialOutput=0  VectorParamsAs1DForOutWhenUnconnected=off
  wires:
  iq/1 -> Sum3/2, Saturation Dynamic/2
  Saturation Dynamic/1 -> Sum3/1
  iq_max/1 -> Saturation Dynamic/1
  iq_min/1 -> Saturation Dynamic/3
  cf_iqKiLimProt/1 -> Divide1/2
  Divide1/1 -> iq_limProtErr/1
  Sum3/1 -> Divide1/1

== system BLDCmotor_FOC_R2017b_fixdt/BLDC_controller/F05_Field_Oriented_Control/Motor_Limitations/Motor_Limitations_Enabled/Torque_Mode_Protection ==
  n_motAbs : Inport
  n_max : Inport  Port=2
  Vq_max : Inport  Port=3
  Action Port : ActionPort  InitializeStates=reset  ActionPortLabel=case [ 3 ]:
  Constant1 : Constant  Value=0  OutDataTypeStr=uint8
  Data Type Conversion2 : DataTypeConversion  Commented=on  OutDataTypeStr=fixdt(0,16,12)  SaturateOnIntegerOverflow=off  RndMeth=Floor
  I_backCalc_fixdt : BLDC_controller_Lib/I_backCalc_fixdt  Commented=on  yInit=0
      settings: AttributesFormatString=Ini=%<yInit>
  PI Controller : slpidlib/PID Controller  Controller=I  Form=Parallel  TimeDomain=Discrete-time  UseExternalTs=on  SampleTime=-1  IntegratorMethod=Forward Euler  FilterMethod=Forward Euler  ControllerParametersSource=external  P=0.6  I=0.05  UseKiTs=on  D=0  UseExternalDerivativeSource=off  N=100  UseFilter=on  TunerSelectOption=Transfer Function Based (PID Tuner App)  ZeroCross=off  InitialConditionSource=external  InitialConditionForIntegrator=0  InitialConditionForFilter=0  DifferentiatorICPrevScaledInput=0  ExternalReset=none  TrackingMode=off  Kt=1  LimitOutput=on  SatLimitsSource=external  UpperSaturationLimit=1  LowerSaturationLimit=-1  LinearizeAsGain=on  AntiWindupMode=back-calculation  Kb=cf_KbLimProt  LimitIntegrator=off  UpperIntegratorSaturationLimit=inf  LowerIntegratorSaturationLimit=-inf  RndMeth=Simplest  SaturateOnIntegerOverflow=on  POutMin=[]  POutMax=[]  IOutMin=[]  IOutMax=[]  DOutMin=[]  DOutMax=[]  NOutMin=[]  NOutMax=[]  SumOutMin=[]  SumOutMax=[]  SaturationOutDataTypeStr=Inherit: Inherit via back propagation  SaturationOutMin=[]  SaturationOutMax=[]  PParamMin=[]  PParamMax=[]  IParamMin=[]  IParamMax=[]  DParamMin=[]  DParamMax=[]  NParamMin=[]  NParamMax=[]  KbParamMin=[]  KbParamMax=[]  KtParamMin=[]  KtParamMax=[]  KbOutMin=[]  KbOutMax=[]  KtOutMin=[]  KtOutMax=[]  IntegratorOutDataTypeStr=Inherit: Inherit via back propagation  IntegratorOutMin=[]  IntegratorOutMax=[]  FilterOutMin=[]  FilterOutMax=[]  SumI1OutMin=[]  SumI1OutMax=[]  SumI2OutMin=[]  SumI2OutMax=[]  SumI3OutMin=[]  SumI3OutMax=[]  SumI4OutMin=[]  SumI4OutMax=[]  SumDOutMin=[]  SumDOutMax=[]  DifferentiatorOutMin=[]  DifferentiatorOutMax=[]  FilterDiffOutCoefMin=[]  FilterDiffOutCoefMax=[]  ReciprocalOutMin=[]  ReciprocalOutMax=[]  SumDenOutMin=[]  SumDenOutMax=[]  SumNumOutMin=[]  SumNumOutMax=[]  DivideOutMin=[]  DivideOutMax=[]  UdiffTsProdOutMin=[]  UdiffTsProdOutMax=[]  NTsProdOutMin=[]  NTsProdOutMax=[]  UintegralTsProdOutMin=[]  UintegralTsProdOutMax=[]  UngainTsProdOutMin=[]  UngainTsProdOutMax=[]  ClampingZeroOutDataTypeStr=Inherit: Inherit via back propagation  ClampingZeroOutMin=[]  ClampingZeroOutMax=[]  FilterDenConstantOutDataTypeStr=Inherit: Inherit via back propagation  FilterDenConstantOutMin=[]  FilterDenConstantOutMax=[]  PCopyOutDataTypeStr=Inherit: Inherit via back propagation  PCopyOutMin=[]  PCopyOutMax=[]  NCopyOutDataTypeStr=Inherit: Inherit via back propagation  NCopyOutMin=[]  NCopyOutMax=[]  IntegratorContinuousStateAttributes=''  IntegratorStateMustResolveToSignalObject=off  IntegratorRTWStateStorageClass=Auto  FilterContinuousStateAttributes=''  FilterStateMustResolveToSignalObject=off  FilterRTWStateStorageClass=Auto  ParallelPVariant=Disabled  IdealPVariant=Disabled  IVariant=ExternalParameters  DVariant=Disabled  IntegratorVariant=Discrete  SatVariant=External  AWVariant=BackCalculation  PCopyVariant=Disabled  TRVariant=Disabled  FdbkBlocksVariant=Forward  IdealPFdbkVariant=Disabled  SatFdbkVariant=Disabled  DerivativeFilterVariant=Disabled  NVariant=Disabled  NCopyVariant=Disabled_SignalSpec  FilterICVariant=Disabled  IntegratorICVariant=ExternalICs  ExternalResetVariant=Disabled  TRSumVariant=Passthrough  SumFdbkVariant=Disabled  SumVariant=Passthrough_I  TsampFilterVariant=InternalTs  TsampNgainVariant=Passthrough  TsampIntegralVariant=Passthrough  ExternalSaturationOutDataTypeStr=Inherit: Same as second input  DerivativeSourceVariant=Disabled  PreIntVariant=InternalPreInt
      settings: LibrarySourceBlock=mcblib/Controls/Controllers/PI Controller
  Sum1 : Sum  Inputs=+-  RndMeth=Simplest
  Variant Subsystem1 : Subsystem  Variant=on  VariantActivationTime=code compile
  cf_KbLimProt : Constant  Commented=on  Value=cf_KbLimProt  OutDataTypeStr=fixdt(0,16,12)
  cf_nKiLimProt : Constant  Value=cf_nKiLimProt  OutDataTypeStr=fixdt(0,16,16)
  Vq_nLimProtMax : Outport  InitialOutput=0  VectorParamsAs1DForOutWhenUnconnected=off
  wires:
  n_motAbs/1 -> [n_motAbs]
  n_max/1 -> [n_max]
  Sum1/1 -> PI Controller/1
  [n_motAbs] -> Sum1/2
  [n_max] -> Sum1/1
  cf_nKiLimProt/1 -> PI Controller/2
  Vq_max/1 -> [Vq_max]
  Constant1/1 -> PI Controller/5
  PI Controller/1 -> Vq_nLimProtMax/1
  [Vq_max] -> PI Controller/4
  cf_KbLimProt/1 -> I_backCalc_fixdt/2
  Variant Subsystem1/1(Vd_max_margin) -> PI Controller/3

== system BLDCmotor_FOC_R2017b_fixdt/BLDC_controller/F05_Field_Oriented_Control/Motor_Limitations/Motor_Limitations_Enabled/Variant Subsystem ==
  note: 1) Add Subsystem or Model blocks as valid variant choices.
      | 2) You cannot connect blocks at this level. At simulation, connectivity is automatically
      | determined, based on the active variant and port name matching.
  VdPrev : Inport
  GD32F103 : Subsystem  TreatAsAtomicUnit=on  VariantControl=mcu_model == 1
  STM32F103 : Subsystem  TreatAsAtomicUnit=on  VariantControl=mcu_model == 0
  Vd_max : Outport
  Vd_min : Outport  Port=2
  Vq_max : Outport  Port=3
  Vq_min : Outport  Port=4

== system BLDCmotor_FOC_R2017b_fixdt/BLDC_controller/F05_Field_Oriented_Control/Motor_Limitations/Motor_Limitations_Enabled/Voltage_Mode_Protection ==
  r_inpTgtScaAbs : Inport
  iqAbs : Inport  Port=2
  iq_max : Inport  Port=3
  n_motAbs : Inport  Port=4
  n_max : Inport  Port=5
  Action Port : ActionPort  InitializeStates=reset  ActionPortLabel=case [ 1 ]:
  Constant : Constant  Value=0  OutDataTypeStr=Inherit: Inherit via back propagation
  Constant1 : Constant  Value=0  OutDataTypeStr=Inherit: Inherit via back propagation
  I_backCalc_fixdt : BLDC_controller_Lib/I_backCalc_fixdt  yInit=1000
      settings: AttributesFormatString=Ini=%<yInit>
  I_backCalc_fixdt1 : BLDC_controller_Lib/I_backCalc_fixdt  yInit=1000
      settings: AttributesFormatString=Ini=%<yInit>
  Sum1 : Sum  Inputs=+-  RndMeth=Simplest  OutDataTypeStr=Inherit: Same as first input
  Sum2 : Sum  Inputs=+-  RndMeth=Simplest  OutDataTypeStr=Inherit: Same as first input
  cf_KbLimProt : Constant  Value=cf_KbLimProt  OutDataTypeStr=fixdt(0,16,12)
  cf_iqKiLimProt : Constant  Value=cf_iqKiLimProt  OutDataTypeStr=fixdt(0,16,16)
  cf_nKiLimProt : Constant  Value=cf_nKiLimProt  OutDataTypeStr=fixdt(0,16,16)
  r_iqLimProtMax : Outport  InitialOutput=0  VectorParamsAs1DForOutWhenUnconnected=off
  r_nLimProtMax : Outport  Port=2  InitialOutput=0  VectorParamsAs1DForOutWhenUnconnected=off
  wires:
  iq_max/1 -> [iq_max]
  iqAbs/1 -> [iqAbs]
  n_max/1 -> [n_max]
  n_motAbs/1 -> [n_motAbs]
  Sum2/1 -> I_backCalc_fixdt/1
  [iq_max] -> Sum2/1
  [iqAbs] -> Sum2/2
  Constant/1 -> I_backCalc_fixdt/5
  [r_inpTgtScaAbs] -> I_backCalc_fixdt1/4, I_backCalc_fixdt/4
  cf_iqKiLimProt/1 -> I_backCalc_fixdt/2
  cf_KbLimProt/1 -> I_backCalc_fixdt1/3, I_backCalc_fixdt/3
  [r_iqLimProtMax] -> r_iqLimProtMax/1
  I_backCalc_fixdt/1 -> [r_iqLimProtMax]
  [r_nLimProtMax] -> r_nLimProtMax/1
  I_backCalc_fixdt1/1 -> [r_nLimProtMax]
  cf_nKiLimProt/1 -> I_backCalc_fixdt1/2
  Constant1/1 -> I_backCalc_fixdt1/5
  [n_motAbs] -> Sum1/2
  [n_max] -> Sum1/1
  Sum1/1 -> I_backCalc_fixdt1/1
  r_inpTgtScaAbs/1 -> [r_inpTgtScaAbs]

== system BLDCmotor_FOC_R2017b_fixdt/BLDC_controller/F03_Control_Mode_Manager/F03_03_Input_Target_Synthesis/FOC_Control_Type/Variant Subsystem1/GD32F103 ==
  Vd_max1 : Constant  Value=GD32_Vd_max_margin  OutDataTypeStr=fixdt(1,16,4)
  Vd_max_margin : Outport
  wires:
  Vd_max1/1 -> Vd_max_margin/1

== system BLDCmotor_FOC_R2017b_fixdt/BLDC_controller/F03_Control_Mode_Manager/F03_03_Input_Target_Synthesis/FOC_Control_Type/Variant Subsystem1/STM32F103 ==
  Vd_max3 : Constant  Value=STM32_Vd_max_margin  OutDataTypeStr=fixdt(1,16,4)
  Vd_max_margin : Outport
  wires:
  Vd_max3/1 -> Vd_max_margin/1
